simulink model "Modulador_de_torque"  (R2021a)
settings: Solver=VariableStepAuto  StartTime=0.0  StopTime=10.0  RelTol=1e-3
undefined symbols (not defined in the file): beq, lambda_m, Ld, Lq, Pp, R0, Rd, Rq, Rs
settings Model: Creator=fhlla  LastModifiedBy=fhlla

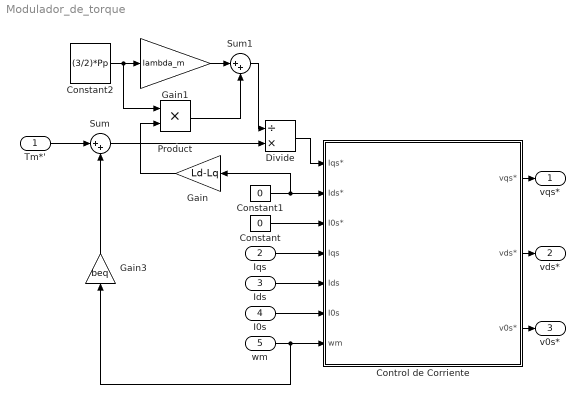
== system Modulador_de_torque ==
  Tm*' : Inport
  Iqs : Inport  Port=2
  Ids : Inport  Port=3
  I0s : Inport  Port=4
  wm : Inport  Port=5
  Constant : Constant  Value=0
  Constant1 : Constant  Value=0
  Constant2 : Constant  Value=(3/2)*Pp
  Control de Corriente : Subsystem
  Divide : Product  Inputs=/*
  Gain : Gain  Gain=Ld-Lq
  Gain1 : Gain  Gain=lambda_m
  Gain3 : Gain  Gain=beq
  Product : Product
  Sum : Sum  Inputs=|++
  Sum1 : Sum  Inputs=|++
  vqs* : Outport
  vds* : Outport  Port=2
  v0s* : Outport  Port=3
  wires:
  Tm*'/1 -> Sum/1
  Constant1/1 -> Gain/1, Control de Corriente/2(Ids*)
  Control de Corriente/1(vqs*) -> vqs*/1
  wm/1 -> Gain3/1, Control de Corriente/7(wm)
  Gain3/1 -> Sum/2
  Constant/1 -> Control de Corriente/3(I0s*)
  Iqs/1 -> Control de Corriente/4(Iqs)
  Ids/1 -> Control de Corriente/5(Ids)
  Control de Corriente/2(vds*) -> vds*/1
  Control de Corriente/3(v0s*) -> v0s*/1
  I0s/1 -> Control de Corriente/6(I0s)
  Gain/1 -> Product/2
  Constant2/1 -> Gain1/1, Product/1
  Gain1/1 -> Sum1/1
  Product/1 -> Sum1/2
  Sum1/1 -> Divide/1
  Sum/1 -> Divide/2
  Divide/1 -> Control de Corriente/1(Iqs*)

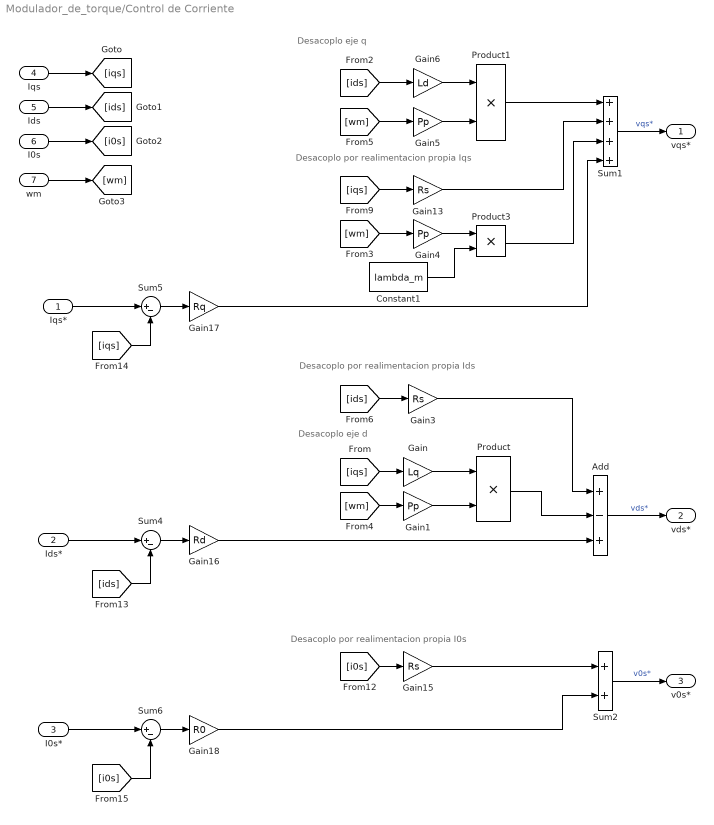
== system Modulador_de_torque/Control de Corriente ==
  note: Desacoplo por realimentacion propia I0s
  note: Desacoplo por realimentacion propia Iqs
  note: Desacoplo por realimentacion propia Ids
  note: Desacoplo eje d
  note: Desacoplo eje q
  Iqs* : Inport
  Ids* : Inport  Port=2
  I0s* : Inport  Port=3
  Iqs : Inport  Port=4
  Ids : Inport  Port=5
  I0s : Inport  Port=6
  wm : Inport  Port=7
  Add : Sum  Inputs=+-+
  Constant1 : Constant  Value=lambda_m
  Gain : Gain  Gain=Lq
  Gain1 : Gain  Gain=Pp
  Gain13 : Gain  Gain=Rs
  Gain15 : Gain  Gain=Rs
  Gain16 : Gain  Gain=Rd
  Gain17 : Gain  Gain=Rq
  Gain18 : Gain  Gain=R0
  Gain3 : Gain  Gain=Rs
  Gain4 : Gain  Gain=Pp
  Gain5 : Gain  Gain=Pp
  Gain6 : Gain  Gain=Ld
  Product : Product
  Product1 : Product
  Product3 : Product
  Sum1 : Sum  Inputs=++++
  Sum2 : Sum
  Sum4 : Sum  Inputs=|+-
  Sum5 : Sum  Inputs=|+-
  Sum6 : Sum  Inputs=|+-
  vqs* : Outport
  vds* : Outport  Port=2
  v0s* : Outport  Port=3
  wires:
  [i0s] -> Sum6/2
  Sum2/1 -> v0s*/1  "v0s*"
  Iqs*/1 -> Sum5/1
  I0s*/1 -> Sum6/1
  [iqs] -> Gain13/1
  [ids] -> Sum4/2
  [i0s] -> Gain15/1
  Sum5/1 -> Gain17/1
  [iqs] -> Sum5/2
  [ids] -> Gain3/1
  Gain13/1 -> Sum1/2
  Sum6/1 -> Gain18/1
  Ids*/1 -> Sum4/1
  Gain15/1 -> Sum2/1
  Gain18/1 -> Sum2/2
  Gain17/1 -> Sum1/4
  Product1/1 -> Sum1/1
  Product/1 -> Add/2
  Gain5/1 -> Product1/2
  Gain/1 -> Product/1
  Gain4/1 -> Product3/1
  Sum4/1 -> Gain16/1
  Constant1/1 -> Product3/2
  Product3/1 -> Sum1/3
  Add/1 -> vds*/1  "vds*"
  Sum1/1 -> vqs*/1  "vqs*"
  Iqs/1 -> [iqs]
  Ids/1 -> [ids]
  I0s/1 -> [i0s]
  [iqs] -> Gain/1
  Gain1/1 -> Product/2
  [wm] -> Gain1/1
  wm/1 -> [wm]
  [wm] -> Gain4/1
  [wm] -> Gain5/1
  [ids] -> Gain6/1
  Gain6/1 -> Product1/1
  Gain16/1 -> Add/3
  Gain3/1 -> Add/1
